simulink model "reaction_wheel_control"  (R2021a)
settings: Solver=VariableStepAuto  StartTime=0.0  StopTime=10.0  RelTol=1e-3
libraries: arduinolib x15, pid_lib x2, arduinosensorlib x1
settings Model: Creator=vikram  LastModifiedBy=vikram

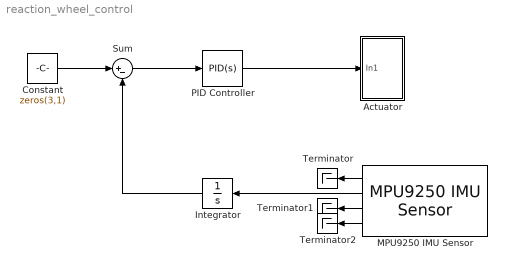
== system reaction_wheel_control ==
  Actuator : Subsystem
  Constant : Constant  Value=zeros(3,1)
  Integrator : Integrator
  MPU9250 IMU Sensor : arduinosensorlib/MPU9250 IMU Sensor  SlaveAddress=0x68  Accel=on  AngularRate=on  Ak8963Field=on  Temperature=on  Status=off  EulerAngles=off  Quat=off  AccelRange=2G  Acceldlpf=218.1 Hz  GyroRange=250 dps  Gyrodlpf=250 Hz  DmpOdr=200 Hz  SampleTime=-1
      settings: SourceProductBaseCode=ARDUINO
  PID Controller : pid_lib/PID Controller  Controller=PID  Form=Parallel  TimeDomain=Continuous-time  UseExternalTs=off  SampleTime=-1  IntegratorMethod=Forward Euler  FilterMethod=Forward Euler  ControllerParametersSource=internal  P=1  I=1  D=0  UseFilter=on  N=100  TunerSelectOption=Transfer Function Based (PID Tuner App)  InitialConditionSource=internal  InitialConditionForIntegrator=0  InitialConditionForFilter=0  DifferentiatorICPrevScaledInput=0  ExternalReset=none  TrackingMode=off  Kt=1  LimitOutput=off  SatLimitsSource=internal  UpperSaturationLimit=inf  LowerSaturationLimit=-inf  LinearizeAsGain=on  AntiWindupMode=none  Kb=1  POutMin=[]  POutMax=[]  IOutMin=[]  IOutMax=[]  DOutMin=[]  DOutMax=[]  NOutMin=[]  NOutMax=[]  SumOutMin=[]  SumOutMax=[]  SaturationOutMin=[]  SaturationOutMax=[]  PParamMin=[]  PParamMax=[]  IParamMin=[]  IParamMax=[]  DParamMin=[]  DParamMax=[]  NParamMin=[]  NParamMax=[]  KbParamMin=[]  KbParamMax=[]  KtParamMin=[]  KtParamMax=[]  KbOutMin=[]  KbOutMax=[]  KtOutMin=[]  KtOutMax=[]  IntegratorOutMin=[]  IntegratorOutMax=[]  FilterOutMin=[]  FilterOutMax=[]  SumI1OutMin=[]  SumI1OutMax=[]  SumI2OutMin=[]  SumI2OutMax=[]  SumI3OutMin=[]  SumI3OutMax=[]  SumI4OutMin=[]  SumI4OutMax=[]  SumDOutMin=[]  SumDOutMax=[]  DifferentiatorOutMin=[]  DifferentiatorOutMax=[]  FilterDiffOutCoefMin=[]  FilterDiffOutCoefMax=[]  ReciprocalOutMin=[]  ReciprocalOutMax=[]  SumDenOutMin=[]  SumDenOutMax=[]  SumNumOutMin=[]  SumNumOutMax=[]  DivideOutMin=[]  DivideOutMax=[]  UdiffTsProdOutMin=[]  UdiffTsProdOutMax=[]  NTsProdOutMin=[]  NTsProdOutMax=[]  UintegralTsProdOutMin=[]  UintegralTsProdOutMax=[]  UngainTsProdOutMin=[]  UngainTsProdOutMax=[]  IntegratorContinuousStateAttributes=''  IntegratorStateMustResolveToSignalObject=off  IntegratorRTWStateStorageClass=Auto  FilterContinuousStateAttributes=''  FilterStateMustResolveToSignalObject=off  FilterRTWStateStorageClass=Auto  ParallelPVariant=InternalParameters  IdealPVariant=Disabled  IVariant=InternalParameters  DVariant=InternalParameters  IntegratorVariant=Continuous  SatVariant=Disabled  AWVariant=Passthrough  PCopyVariant=Disabled  TRVariant=Disabled  FdbkBlocksVariant=Forward  IdealPFdbkVariant=Disabled  SatFdbkVariant=Disabled  DerivativeFilterVariant=ContFilter  NVariant=InternalParameters  NCopyVariant=Disabled  FilterICVariant=InternalICsFilter  IntegratorICVariant=InternalICs  ExternalResetVariant=Disabled  TRSumVariant=Passthrough  SumFdbkVariant=Disabled  SumVariant=Sum_PID  TsampFilterVariant=InternalTs  TsampNgainVariant=Passthrough  TsampIntegralVariant=Passthrough  ExternalSaturationOutDataTypeStr=Inherit: Same as second input
  Sum : Sum  Inputs=|+-
  Terminator : Terminator
  Terminator1 : Terminator
  Terminator2 : Terminator
  wires:
  MPU9250 IMU Sensor/1 -> Terminator/1
  MPU9250 IMU Sensor/3 -> Terminator1/1
  MPU9250 IMU Sensor/4 -> Terminator2/1
  MPU9250 IMU Sensor/2 -> Integrator/1
  PID Controller/1 -> Actuator/1(In1)
  Integrator/1 -> Sum/2
  Sum/1 -> PID Controller/1
  Constant/1 -> Sum/1

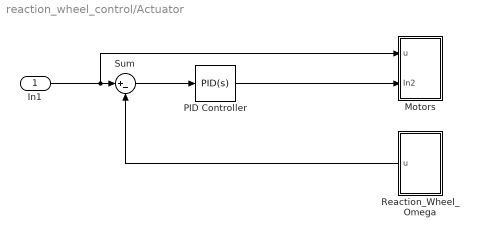
== system reaction_wheel_control/Actuator ==
  In1 : Inport
  Motors : Subsystem
  PID Controller : pid_lib/PID Controller  Controller=PID  Form=Parallel  TimeDomain=Continuous-time  UseExternalTs=off  SampleTime=-1  IntegratorMethod=Forward Euler  FilterMethod=Forward Euler  ControllerParametersSource=internal  P=1  I=1  D=0  UseFilter=on  N=100  TunerSelectOption=Transfer Function Based (PID Tuner App)  InitialConditionSource=internal  InitialConditionForIntegrator=0  InitialConditionForFilter=0  DifferentiatorICPrevScaledInput=0  ExternalReset=none  TrackingMode=off  Kt=1  LimitOutput=off  SatLimitsSource=internal  UpperSaturationLimit=inf  LowerSaturationLimit=-inf  LinearizeAsGain=on  AntiWindupMode=none  Kb=1  POutMin=[]  POutMax=[]  IOutMin=[]  IOutMax=[]  DOutMin=[]  DOutMax=[]  NOutMin=[]  NOutMax=[]  SumOutMin=[]  SumOutMax=[]  SaturationOutMin=[]  SaturationOutMax=[]  PParamMin=[]  PParamMax=[]  IParamMin=[]  IParamMax=[]  DParamMin=[]  DParamMax=[]  NParamMin=[]  NParamMax=[]  KbParamMin=[]  KbParamMax=[]  KtParamMin=[]  KtParamMax=[]  KbOutMin=[]  KbOutMax=[]  KtOutMin=[]  KtOutMax=[]  IntegratorOutMin=[]  IntegratorOutMax=[]  FilterOutMin=[]  FilterOutMax=[]  SumI1OutMin=[]  SumI1OutMax=[]  SumI2OutMin=[]  SumI2OutMax=[]  SumI3OutMin=[]  SumI3OutMax=[]  SumI4OutMin=[]  SumI4OutMax=[]  SumDOutMin=[]  SumDOutMax=[]  DifferentiatorOutMin=[]  DifferentiatorOutMax=[]  FilterDiffOutCoefMin=[]  FilterDiffOutCoefMax=[]  ReciprocalOutMin=[]  ReciprocalOutMax=[]  SumDenOutMin=[]  SumDenOutMax=[]  SumNumOutMin=[]  SumNumOutMax=[]  DivideOutMin=[]  DivideOutMax=[]  UdiffTsProdOutMin=[]  UdiffTsProdOutMax=[]  NTsProdOutMin=[]  NTsProdOutMax=[]  UintegralTsProdOutMin=[]  UintegralTsProdOutMax=[]  UngainTsProdOutMin=[]  UngainTsProdOutMax=[]  IntegratorContinuousStateAttributes=''  IntegratorStateMustResolveToSignalObject=off  IntegratorRTWStateStorageClass=Auto  FilterContinuousStateAttributes=''  FilterStateMustResolveToSignalObject=off  FilterRTWStateStorageClass=Auto  ParallelPVariant=InternalParameters  IdealPVariant=Disabled  IVariant=InternalParameters  DVariant=InternalParameters  IntegratorVariant=Continuous  SatVariant=Disabled  AWVariant=Passthrough  PCopyVariant=Disabled  TRVariant=Disabled  FdbkBlocksVariant=Forward  IdealPFdbkVariant=Disabled  SatFdbkVariant=Disabled  DerivativeFilterVariant=ContFilter  NVariant=InternalParameters  NCopyVariant=Disabled  FilterICVariant=InternalICsFilter  IntegratorICVariant=InternalICs  ExternalResetVariant=Disabled  TRSumVariant=Passthrough  SumFdbkVariant=Disabled  SumVariant=Sum_PID  TsampFilterVariant=InternalTs  TsampNgainVariant=Passthrough  TsampIntegralVariant=Passthrough  ExternalSaturationOutDataTypeStr=Inherit: Same as second input
  Reaction_Wheel_Omega : Subsystem
  Sum : Sum  Inputs=|+-
  wires:
  In1/1 -> Motors/1(u), Sum/1
  PID Controller/1 -> Motors/2(In2)
  Sum/1 -> PID Controller/1
  Reaction_Wheel_Omega/1(u) -> Sum/2

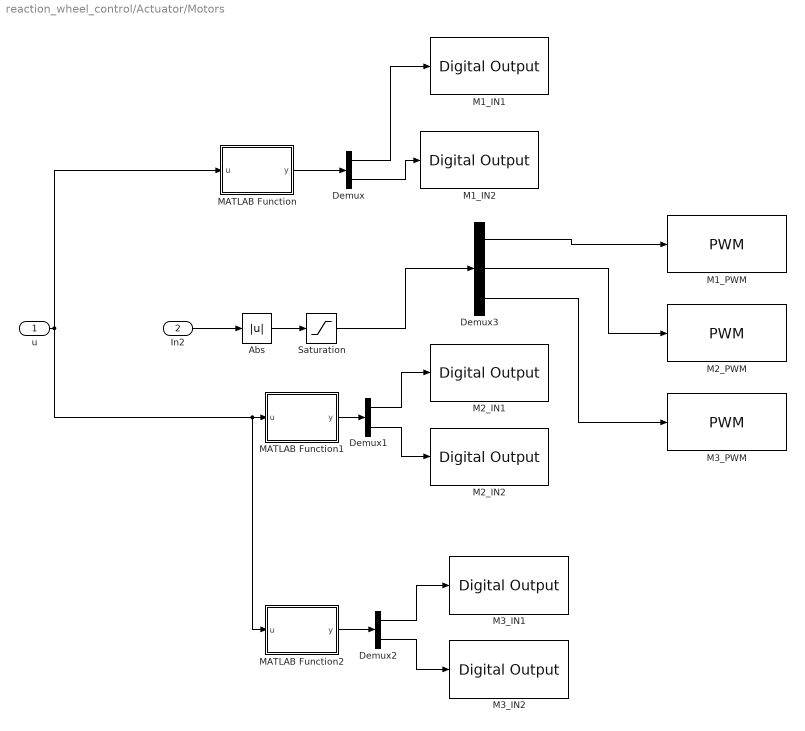
== system reaction_wheel_control/Actuator/Motors ==
  u : Inport
  In2 : Inport  Port=2
  Abs : Abs
  Demux : Demux  Outputs=2
  Demux1 : Demux  Outputs=2
  Demux2 : Demux  Outputs=2
  Demux3 : Demux  Outputs=3
  M1_IN1 : arduinolib/Digital Output  pinNumber=9  Direction=output  blockPlatform=arduino
  M1_IN2 : arduinolib/Digital Output  pinNumber=9  Direction=output  blockPlatform=arduino
  M1_PWM : arduinolib/PWM  pinNumber=5  frequencyType=Default  desiredFrequency=490.2  achievableFrequency=490.2
  M2_IN1 : arduinolib/Digital Output  pinNumber=9  Direction=output  blockPlatform=arduino
  M2_IN2 : arduinolib/Digital Output  pinNumber=9  Direction=output  blockPlatform=arduino
  M2_PWM : arduinolib/PWM  pinNumber=5  frequencyType=Default  desiredFrequency=490.2  achievableFrequency=490.2
  M3_IN1 : arduinolib/Digital Output  pinNumber=9  Direction=output  blockPlatform=arduino
  M3_IN2 : arduinolib/Digital Output  pinNumber=9  Direction=output  blockPlatform=arduino
  M3_PWM : arduinolib/PWM  pinNumber=5  frequencyType=Default  desiredFrequency=490.2  achievableFrequency=490.2
  MATLAB Function : MATLAB Function  TreatAsAtomicUnit=on
  MATLAB Function1 : MATLAB Function  TreatAsAtomicUnit=on
  MATLAB Function2 : MATLAB Function  TreatAsAtomicUnit=on
  Saturation : Saturate  UpperLimit=255  LowerLimit=0
  wires:
  Demux/1 -> M1_IN1/1
  Abs/1 -> Saturation/1
  MATLAB Function1/1(y) -> Demux1/1
  Demux2/1 -> M3_IN1/1
  Demux1/2 -> M2_IN2/1
  Demux/2 -> M1_IN2/1
  MATLAB Function/1(y) -> Demux/1
  MATLAB Function2/1(y) -> Demux2/1
  Demux3/2 -> M2_PWM/1
  Demux2/2 -> M3_IN2/1
  Demux3/3 -> M3_PWM/1
  Saturation/1 -> Demux3/1
  Demux3/1 -> M1_PWM/1
  Demux1/1 -> M2_IN1/1
  u/1 -> MATLAB Function/1(u), MATLAB Function2/1(u), MATLAB Function1/1(u)
  In2/1 -> Abs/1

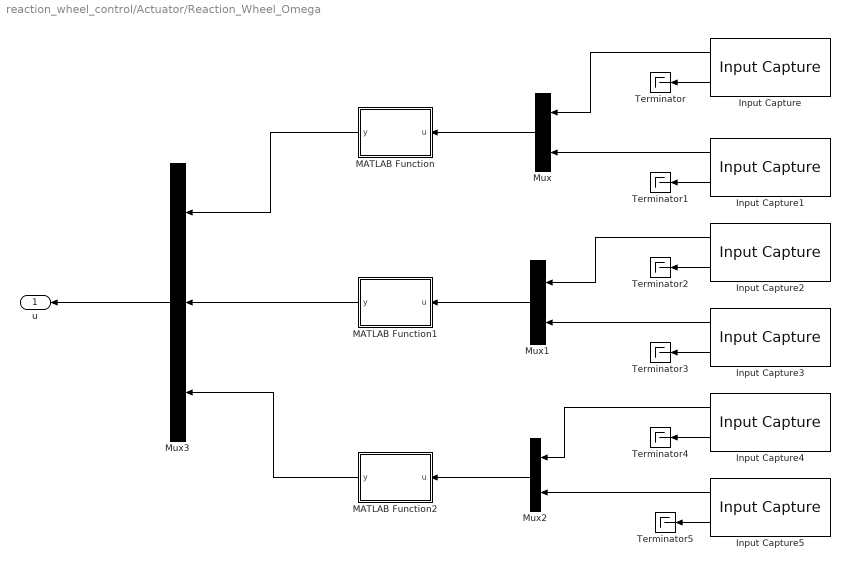
== system reaction_wheel_control/Actuator/Reaction_Wheel_Omega ==
  Input Capture{,1..5} (6 alike) : arduinolib/Input Capture  InputCapturePinNumber=48  SampleTime=0.1
      settings: SourceProductBaseCode=ARDUINO
  MATLAB Function : MATLAB Function  TreatAsAtomicUnit=on
  MATLAB Function1 : MATLAB Function  TreatAsAtomicUnit=on
  MATLAB Function2 : MATLAB Function  TreatAsAtomicUnit=on
  Mux : Mux  Inputs=2
  Mux1 : Mux  Inputs=2
  Mux2 : Mux  Inputs=2
  Mux3 : Mux  Inputs=3
  Terminator{,1..5} (6 alike) : Terminator
  u : Outport
  wires:
  Input Capture/2 -> Terminator/1
  Input Capture1/2 -> Terminator1/1
  Input Capture2/2 -> Terminator2/1
  Input Capture3/2 -> Terminator3/1
  Input Capture4/2 -> Terminator4/1
  Input Capture5/2 -> Terminator5/1
  Input Capture/1 -> Mux/1
  Input Capture1/1 -> Mux/2
  Input Capture2/1 -> Mux1/1
  Input Capture3/1 -> Mux1/2
  Input Capture4/1 -> Mux2/1
  Input Capture5/1 -> Mux2/2
  Mux/1 -> MATLAB Function/1(u)
  Mux1/1 -> MATLAB Function1/1(u)
  Mux2/1 -> MATLAB Function2/1(u)
  MATLAB Function/1(y) -> Mux3/1
  MATLAB Function1/1(y) -> Mux3/2
  MATLAB Function2/1(y) -> Mux3/3
  Mux3/1 -> u/1

== matlab function reaction_wheel_control/Actuator/Reaction_Wheel_Omega/MATLAB Function ==
  data: u input; y output
function y = fcn(u)
global omega_w1
if u(1)>0
    omega_w1=u(1)*2*pi/7;
else
    omega_w1=-u(2)*2*pi/7;
end
y = omega_w1;

== matlab function reaction_wheel_control/Actuator/Reaction_Wheel_Omega/MATLAB Function2 ==
  data: u input; y output
function y = fcn(u)
global omega_w3
if u(1)>0
    omega_w3=u(1)*2*pi/7;
else
    omega_w3=-u(2)*2*pi/7;
end
y = omega_w3;

== matlab function reaction_wheel_control/Actuator/Motors/MATLAB Function ==
  data: u input; y output
function y = fcn(u)
global m1

if u(1)>0
    m1(1)=1;
    m1(2)=-1;
else
    m1(1)=-1;
    m1(2)=1;  
end


y = m1;

== matlab function reaction_wheel_control/Actuator/Motors/MATLAB Function1 ==
  data: u input; y output
function y = fcn(u)
global m2

if u(2)>0
    m2(1)=1;
    m2(2)=-1;
else
    m2(1)=-1;
    m2(2)=1;  
end


y = m2;

== matlab function reaction_wheel_control/Actuator/Motors/MATLAB Function2 ==
  data: u input; y output
function y = fcn(u)
global m3

if u(2)>0
    m3(1)=1;
    m3(2)=-1;
else
    m3(1)=-1;
    m3(2)=1;  
end


y = m3;

== matlab function reaction_wheel_control/Actuator/Reaction_Wheel_Omega/MATLAB Function1 ==
  data: u input; y output
function y = fcn(u)
global omega_w2
if u(1)>0
    omega_w2=u(1)*2*pi/7;
else
    omega_w2=-u(2)*2*pi/7;
end
y = omega_w2;
